simulink model "model_uloha10"  (R2019b)
settings: Solver=VariableStepAuto  StartTime=0.0  StopTime=10.0  RelTol=1e-3
settings Model: Creator=Já  LastModifiedBy=Já

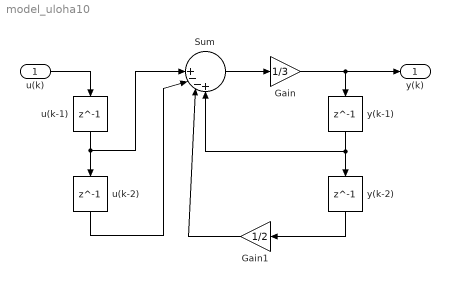
== system model_uloha10 ==
  u(k) : Inport
  Gain : Gain  Gain=1/3
  Gain1 : Gain  Gain=1/2
  Sum : Sum  Inputs=|||+--+
  u(k-1) : Delay  DelayLength=1
  u(k-2) : Delay  DelayLength=1
  y(k-1) : Delay  DelayLength=1
  y(k-2) : Delay  DelayLength=1
  y(k) : Outport
  wires:
  u(k)/1 -> u(k-1)/1
  u(k-1)/1 -> Sum/1, u(k-2)/1
  y(k-1)/1 -> Sum/4, y(k-2)/1
  Gain/1 -> y(k-1)/1, y(k)/1
  Sum/1 -> Gain/1
  y(k-2)/1 -> Gain1/1
  Gain1/1 -> Sum/3
  u(k-2)/1 -> Sum/2
